simulink model "wlan_mac_hw"  (Simulink 7.8)
settings: Solver=ode45  StartTime=0.0  StopTime=200  RelTol=1e-3
PostLoadFcn:
  | wlan_mac_hw_init
InitFcn:
  | wlan_mac_hw_init
StartFcn:
  | wlan_mac_hw_init
values from neighbouring files (symbols this model uses):
  NB_CNTR_NAV = ceil(log2(MAX_NAV * 160))    [wlan_mac_hw_init.m]
  ticks_per_usec = 10    [wlan_mac_hw_init.m]
undefined symbols (not defined in the file or in its folder): gcbh, xlBlockLoadCallback, xlGetNormalizedPeriod
libraries: xbsIndex_r4 x788, xbsEDKLib_r4 x1
(part 5 of 6)

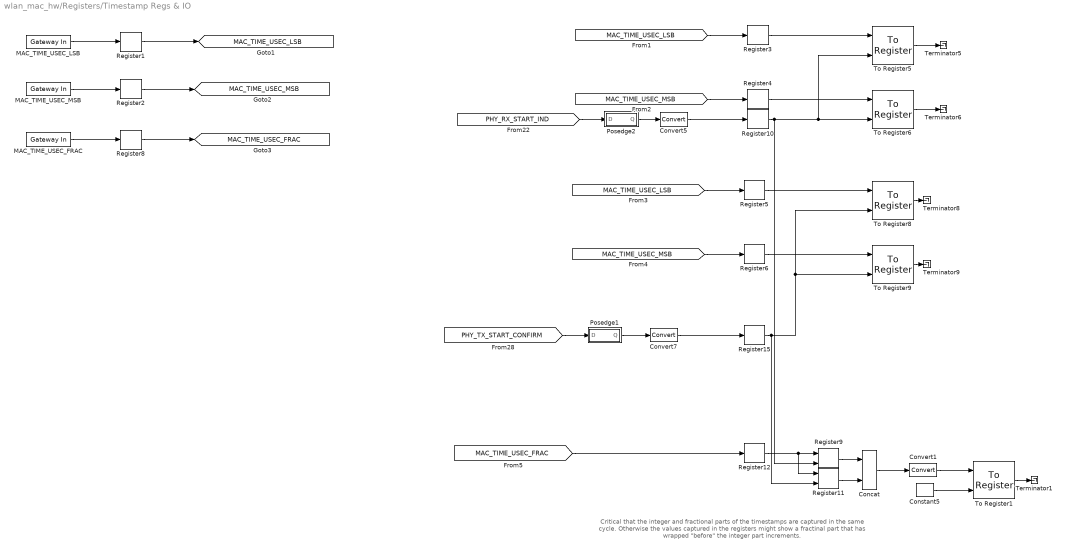
== system wlan_mac_hw/Registers/Timestamp Regs & IO ==
  note: Critical that the integer and fractional parts of the timestamps
      | are captured in the same cycle. Otherwise the values captured in the registers
      | might show a fractinal part that has wrapped "before" the integer part
      | increments.
  Concat : xbsIndex_r4/Concat  num_inputs=2  dbl_ovrd=off  block_type=concat
  Constant5 : xbsIndex_r4/Constant  const=1  gui_display_data_type=Boolean  arith_type=Boolean  n_bits=30  bin_pt=0  preci_type=Single  exp_width=8  frac_width=24  explicit_period=on  period=1  equ=P=C  opselect=C  inp2=PCIN>>17  opr=+  inp1=P  carry=CIN  dbl_ovrd=off  block_type=constant
  Convert1 : xbsIndex_r4/Convert  gui_display_data_type=Fixed-point  arith_type=Unsigned  n_bits=32  bin_pt=0  float_type=Single  exp_bits=8  fraction_bits=24  quantization=Truncate  overflow=Wrap  en=off  latency=0  dbl_ovrd=off  pipeline=off  block_type=convert
  Convert5 : xbsIndex_r4/Convert  gui_display_data_type=Boolean  arith_type=Boolean  n_bits=32  bin_pt=0  float_type=Single  exp_bits=8  fraction_bits=24  quantization=Truncate  overflow=Wrap  en=off  latency=0  dbl_ovrd=off  pipeline=off  block_type=convert
  Convert7 : xbsIndex_r4/Convert  gui_display_data_type=Boolean  arith_type=Boolean  n_bits=32  bin_pt=0  float_type=Single  exp_bits=8  fraction_bits=24  quantization=Truncate  overflow=Wrap  en=off  latency=0  dbl_ovrd=off  pipeline=off  block_type=convert
  MAC_TIME_USEC_FRAC : xbsIndex_r4/Gateway In  gui_display_data_type=Fixed-point  arith_type=Unsigned  n_bits=8  bin_pt=0  preci_type=Single  exp_width=8  frac_width=24  quantization="Round  (unbiased: +/- Inf)"  overflow=Saturate  period=1  dbl_ovrd=off  timing_constraint=None  locs_specified=off  LOCs={}  UseAsADC=off  ADCChannel='1'  inherit_from_input=off  hdl_port=on  block_type=gatewayin
  MAC_TIME_USEC_LSB : xbsIndex_r4/Gateway In  gui_display_data_type=Fixed-point  arith_type=Unsigned  n_bits=32  bin_pt=0  preci_type=Single  exp_width=8  frac_width=24  quantization="Round  (unbiased: +/- Inf)"  overflow=Saturate  period=1  dbl_ovrd=off  timing_constraint=None  locs_specified=off  LOCs={}  UseAsADC=off  ADCChannel='1'  inherit_from_input=off  hdl_port=on  block_type=gatewayin
  MAC_TIME_USEC_MSB : xbsIndex_r4/Gateway In  gui_display_data_type=Fixed-point  arith_type=Unsigned  n_bits=32  bin_pt=0  preci_type=Single  exp_width=8  frac_width=24  quantization="Round  (unbiased: +/- Inf)"  overflow=Saturate  period=1  dbl_ovrd=off  timing_constraint=None  locs_specified=off  LOCs={}  UseAsADC=off  ADCChannel='1'  inherit_from_input=off  hdl_port=on  block_type=gatewayin
  Posedge1 : Subsystem
  Posedge2 : Subsystem
  Register{1..6,8,10,12,15} (10 alike) : xbsIndex_r4/Register  init=0  rst=off  en=off  dbl_ovrd=off  block_type=register
  Register11 : xbsIndex_r4/Register  init=0  rst=off  en=on  dbl_ovrd=off  block_type=register
  Register9 : xbsIndex_r4/Register  init=0  rst=off  en=on  dbl_ovrd=off  block_type=register
  Terminator{1,5..6,8..9} (5 alike) : Terminator
  To Register1 : xbsIndex_r4/To Register  shared_memory_name='TXRX_START_TIMESTAMPS_FRAC'  init=0  ownership=Locally owned and initialized  explicit_data_type=on  gui_display_data_type=Fixed-point  arith_type=Unsigned  n_bits=32  bin_pt=0  preci_type=Single  dbl_ovrd=off  block_type=toreg
      settings: AttributesFormatString=<< %<shared_memory_name> >>  infoedit="Register block that writes data to a shared memory register.  Delay of one sample period."
  To Register5 : xbsIndex_r4/To Register  shared_memory_name='RX_START_TIMESTAMP_LSB'  init=0  ownership=Locally owned and initialized  explicit_data_type=on  gui_display_data_type=Fixed-point  arith_type=Unsigned  n_bits=32  bin_pt=0  preci_type=Single  dbl_ovrd=off  block_type=toreg
      settings: AttributesFormatString=<< %<shared_memory_name> >>  infoedit="Register block that writes data to a shared memory register.  Delay of one sample period."
  To Register6 : xbsIndex_r4/To Register  shared_memory_name='RX_START_TIMESTAMP_MSB'  init=0  ownership=Locally owned and initialized  explicit_data_type=on  gui_display_data_type=Fixed-point  arith_type=Unsigned  n_bits=32  bin_pt=0  preci_type=Single  dbl_ovrd=off  block_type=toreg
      settings: AttributesFormatString=<< %<shared_memory_name> >>  infoedit="Register block that writes data to a shared memory register.  Delay of one sample period."
  To Register8 : xbsIndex_r4/To Register  shared_memory_name='TX_START_TIMESTAMP_LSB'  init=0  ownership=Locally owned and initialized  explicit_data_type=on  gui_display_data_type=Fixed-point  arith_type=Unsigned  n_bits=32  bin_pt=0  preci_type=Single  dbl_ovrd=off  block_type=toreg
      settings: AttributesFormatString=<< %<shared_memory_name> >>  infoedit="Register block that writes data to a shared memory register.  Delay of one sample period."
  To Register9 : xbsIndex_r4/To Register  shared_memory_name='TX_START_TIMESTAMP_MSB'  init=0  ownership=Locally owned and initialized  explicit_data_type=on  gui_display_data_type=Fixed-point  arith_type=Unsigned  n_bits=32  bin_pt=0  preci_type=Single  dbl_ovrd=off  block_type=toreg
      settings: AttributesFormatString=<< %<shared_memory_name> >>  infoedit="Register block that writes data to a shared memory register.  Delay of one sample period."
  tag scope: MAC_TIME_USEC_FRAC=global, MAC_TIME_USEC_LSB=global, MAC_TIME_USEC_MSB=global
  wires:
  [MAC_TIME_USEC_LSB] -> Register3/1
  [PHY_RX_START_IND] -> Posedge2/1(D)
  [MAC_TIME_USEC_MSB] -> Register4/1
  To Register5/1 -> Terminator5/1
  To Register6/1 -> Terminator6/1
  [PHY_TX_START_CONFIRM] -> Posedge1/1(D)
  To Register8/1 -> Terminator8/1
  To Register9/1 -> Terminator9/1
  Register15/1 -> Register11/2, To Register9/2, To Register8/2
  Posedge2/1(Q) -> Convert5/1
  Convert7/1 -> Register15/1
  MAC_TIME_USEC_LSB/1 -> Register1/1
  MAC_TIME_USEC_MSB/1 -> Register2/1
  Register1/1 -> [MAC_TIME_USEC_LSB]
  Register2/1 -> [MAC_TIME_USEC_MSB]
  Register3/1 -> To Register5/1
  Register4/1 -> To Register6/1
  Convert5/1 -> Register10/1
  [MAC_TIME_USEC_LSB] -> Register5/1
  [MAC_TIME_USEC_MSB] -> Register6/1
  Register5/1 -> To Register8/1
  Register6/1 -> To Register9/1
  Posedge1/1(Q) -> Convert7/1
  MAC_TIME_USEC_FRAC/1 -> Register8/1
  Register8/1 -> [MAC_TIME_USEC_FRAC]
  Concat/1 -> Convert1/1
  Register9/1 -> Concat/1
  Register11/1 -> Concat/2
  [MAC_TIME_USEC_FRAC] -> Register12/1
  Convert1/1 -> To Register1/1
  Constant5/1 -> To Register1/2
  To Register1/1 -> Terminator1/1
  Register10/1 -> To Register6/2, To Register5/2, Register9/2
  Register12/1 -> Register9/1, Register11/1

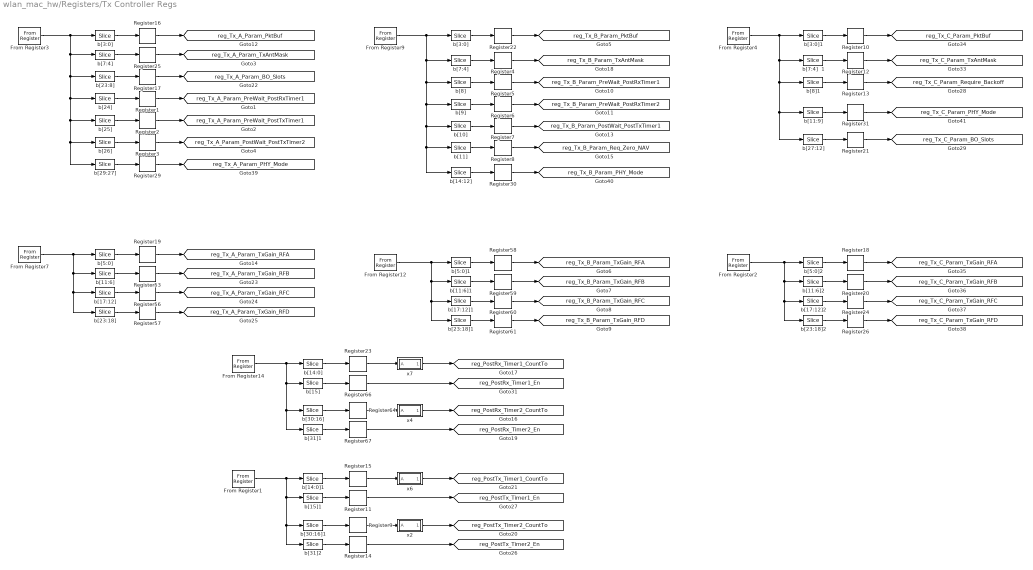
== system wlan_mac_hw/Registers/Tx Controller Regs ==
  " b[10]" : xbsIndex_r4/Slice  nbits=1  boolean_output=on  mode=Lower Bit Location + Width  bit1=0  base1=MSB of Input  bit0=10  base0=LSB of Input  dbl_ovrd=off  block_type=slice
      settings: block_version=VER_STRING_GOES_HERE
  " b[11:6]" : xbsIndex_r4/Slice  nbits=6  boolean_output=off  mode=Lower Bit Location + Width  bit1=0  base1=MSB of Input  bit0=6  base0=LSB of Input  dbl_ovrd=off  block_type=slice
      settings: block_version=VER_STRING_GOES_HERE
  " b[11:6]1" : xbsIndex_r4/Slice  nbits=6  boolean_output=off  mode=Lower Bit Location + Width  bit1=0  base1=MSB of Input  bit0=6  base0=LSB of Input  dbl_ovrd=off  block_type=slice
      settings: block_version=VER_STRING_GOES_HERE
  " b[11:6]2" : xbsIndex_r4/Slice  nbits=6  boolean_output=off  mode=Lower Bit Location + Width  bit1=0  base1=MSB of Input  bit0=6  base0=LSB of Input  dbl_ovrd=off  block_type=slice
      settings: block_version=VER_STRING_GOES_HERE
  " b[11:9]" : xbsIndex_r4/Slice  nbits=3  boolean_output=off  mode=Lower Bit Location + Width  bit1=0  base1=MSB of Input  bit0=9  base0=LSB of Input  dbl_ovrd=off  block_type=slice
      settings: block_version=VER_STRING_GOES_HERE
  " b[11]" : xbsIndex_r4/Slice  nbits=1  boolean_output=on  mode=Lower Bit Location + Width  bit1=0  base1=MSB of Input  bit0=11  base0=LSB of Input  dbl_ovrd=off  block_type=slice
      settings: block_version=VER_STRING_GOES_HERE
  " b[14:0]" : xbsIndex_r4/Slice  nbits=15  boolean_output=off  mode=Lower Bit Location + Width  bit1=0  base1=MSB of Input  bit0=0  base0=LSB of Input  dbl_ovrd=off  block_type=slice
      settings: block_version=VER_STRING_GOES_HERE
  " b[14:0]1" : xbsIndex_r4/Slice  nbits=15  boolean_output=off  mode=Lower Bit Location + Width  bit1=0  base1=MSB of Input  bit0=0  base0=LSB of Input  dbl_ovrd=off  block_type=slice
      settings: block_version=VER_STRING_GOES_HERE
  " b[14:12]" : xbsIndex_r4/Slice  nbits=3  boolean_output=off  mode=Lower Bit Location + Width  bit1=0  base1=MSB of Input  bit0=12  base0=LSB of Input  dbl_ovrd=off  block_type=slice
      settings: block_version=VER_STRING_GOES_HERE
  " b[15]" : xbsIndex_r4/Slice  nbits=1  boolean_output=on  mode=Lower Bit Location + Width  bit1=0  base1=MSB of Input  bit0=15  base0=LSB of Input  dbl_ovrd=off  block_type=slice
      settings: block_version=VER_STRING_GOES_HERE
  " b[15]1" : xbsIndex_r4/Slice  nbits=1  boolean_output=on  mode=Lower Bit Location + Width  bit1=0  base1=MSB of Input  bit0=15  base0=LSB of Input  dbl_ovrd=off  block_type=slice
      settings: block_version=VER_STRING_GOES_HERE
  " b[17:12]" : xbsIndex_r4/Slice  nbits=6  boolean_output=off  mode=Lower Bit Location + Width  bit1=0  base1=MSB of Input  bit0=12  base0=LSB of Input  dbl_ovrd=off  block_type=slice
      settings: block_version=VER_STRING_GOES_HERE
  " b[17:12]1" : xbsIndex_r4/Slice  nbits=6  boolean_output=off  mode=Lower Bit Location + Width  bit1=0  base1=MSB of Input  bit0=12  base0=LSB of Input  dbl_ovrd=off  block_type=slice
      settings: block_version=VER_STRING_GOES_HERE
  " b[17:12]2" : xbsIndex_r4/Slice  nbits=6  boolean_output=off  mode=Lower Bit Location + Width  bit1=0  base1=MSB of Input  bit0=12  base0=LSB of Input  dbl_ovrd=off  block_type=slice
      settings: block_version=VER_STRING_GOES_HERE
  " b[23:18]" : xbsIndex_r4/Slice  nbits=6  boolean_output=off  mode=Lower Bit Location + Width  bit1=0  base1=MSB of Input  bit0=18  base0=LSB of Input  dbl_ovrd=off  block_type=slice
      settings: block_version=VER_STRING_GOES_HERE
  " b[23:18]1" : xbsIndex_r4/Slice  nbits=6  boolean_output=off  mode=Lower Bit Location + Width  bit1=0  base1=MSB of Input  bit0=18  base0=LSB of Input  dbl_ovrd=off  block_type=slice
      settings: block_version=VER_STRING_GOES_HERE
  " b[23:18]2" : xbsIndex_r4/Slice  nbits=6  boolean_output=off  mode=Lower Bit Location + Width  bit1=0  base1=MSB of Input  bit0=18  base0=LSB of Input  dbl_ovrd=off  block_type=slice
      settings: block_version=VER_STRING_GOES_HERE
  " b[23:8]" : xbsIndex_r4/Slice  nbits=16  boolean_output=off  mode=Lower Bit Location + Width  bit1=0  base1=MSB of Input  bit0=8  base0=LSB of Input  dbl_ovrd=off  block_type=slice
      settings: block_version=VER_STRING_GOES_HERE
  " b[24]" : xbsIndex_r4/Slice  nbits=1  boolean_output=on  mode=Lower Bit Location + Width  bit1=0  base1=MSB of Input  bit0=24  base0=LSB of Input  dbl_ovrd=off  block_type=slice
      settings: block_version=VER_STRING_GOES_HERE
  " b[25]" : xbsIndex_r4/Slice  nbits=1  boolean_output=on  mode=Lower Bit Location + Width  bit1=0  base1=MSB of Input  bit0=25  base0=LSB of Input  dbl_ovrd=off  block_type=slice
      settings: block_version=VER_STRING_GOES_HERE
  " b[26]" : xbsIndex_r4/Slice  nbits=1  boolean_output=on  mode=Lower Bit Location + Width  bit1=0  base1=MSB of Input  bit0=26  base0=LSB of Input  dbl_ovrd=off  block_type=slice
      settings: block_version=VER_STRING_GOES_HERE
  " b[27:12]" : xbsIndex_r4/Slice  nbits=16  boolean_output=off  mode=Lower Bit Location + Width  bit1=0  base1=MSB of Input  bit0=12  base0=LSB of Input  dbl_ovrd=off  block_type=slice
      settings: block_version=VER_STRING_GOES_HERE
  " b[29:27]" : xbsIndex_r4/Slice  nbits=3  boolean_output=off  mode=Lower Bit Location + Width  bit1=0  base1=MSB of Input  bit0=27  base0=LSB of Input  dbl_ovrd=off  block_type=slice
      settings: block_version=VER_STRING_GOES_HERE
  " b[30:16]" : xbsIndex_r4/Slice  nbits=15  boolean_output=off  mode=Lower Bit Location + Width  bit1=0  base1=MSB of Input  bit0=16  base0=LSB of Input  dbl_ovrd=off  block_type=slice
      settings: block_version=VER_STRING_GOES_HERE
  " b[30:16]1" : xbsIndex_r4/Slice  nbits=15  boolean_output=off  mode=Lower Bit Location + Width  bit1=0  base1=MSB of Input  bit0=16  base0=LSB of Input  dbl_ovrd=off  block_type=slice
      settings: block_version=VER_STRING_GOES_HERE
  " b[31]1" : xbsIndex_r4/Slice  nbits=1  boolean_output=on  mode=Lower Bit Location + Width  bit1=0  base1=MSB of Input  bit0=31  base0=LSB of Input  dbl_ovrd=off  block_type=slice
      settings: block_version=VER_STRING_GOES_HERE
  " b[31]2" : xbsIndex_r4/Slice  nbits=1  boolean_output=on  mode=Lower Bit Location + Width  bit1=0  base1=MSB of Input  bit0=31  base0=LSB of Input  dbl_ovrd=off  block_type=slice
      settings: block_version=VER_STRING_GOES_HERE
  " b[3:0]" : xbsIndex_r4/Slice  nbits=4  boolean_output=off  mode=Lower Bit Location + Width  bit1=0  base1=MSB of Input  bit0=0  base0=LSB of Input  dbl_ovrd=off  block_type=slice
      settings: block_version=VER_STRING_GOES_HERE
  " b[3:0] " : xbsIndex_r4/Slice  nbits=4  boolean_output=off  mode=Lower Bit Location + Width  bit1=0  base1=MSB of Input  bit0=0  base0=LSB of Input  dbl_ovrd=off  block_type=slice
      settings: block_version=VER_STRING_GOES_HERE
  " b[3:0]1" : xbsIndex_r4/Slice  nbits=4  boolean_output=off  mode=Lower Bit Location + Width  bit1=0  base1=MSB of Input  bit0=0  base0=LSB of Input  dbl_ovrd=off  block_type=slice
      settings: block_version=VER_STRING_GOES_HERE
  " b[5:0]" : xbsIndex_r4/Slice  nbits=6  boolean_output=off  mode=Lower Bit Location + Width  bit1=0  base1=MSB of Input  bit0=0  base0=LSB of Input  dbl_ovrd=off  block_type=slice
      settings: block_version=VER_STRING_GOES_HERE
  " b[5:0]1" : xbsIndex_r4/Slice  nbits=6  boolean_output=off  mode=Lower Bit Location + Width  bit1=0  base1=MSB of Input  bit0=0  base0=LSB of Input  dbl_ovrd=off  block_type=slice
      settings: block_version=VER_STRING_GOES_HERE
  " b[5:0]2" : xbsIndex_r4/Slice  nbits=6  boolean_output=off  mode=Lower Bit Location + Width  bit1=0  base1=MSB of Input  bit0=0  base0=LSB of Input  dbl_ovrd=off  block_type=slice
      settings: block_version=VER_STRING_GOES_HERE
  " b[7:4]" : xbsIndex_r4/Slice  nbits=4  boolean_output=off  mode=Lower Bit Location + Width  bit1=0  base1=MSB of Input  bit0=4  base0=LSB of Input  dbl_ovrd=off  block_type=slice
      settings: block_version=VER_STRING_GOES_HERE
  " b[7:4]  " : xbsIndex_r4/Slice  nbits=4  boolean_output=off  mode=Lower Bit Location + Width  bit1=0  base1=MSB of Input  bit0=4  base0=LSB of Input  dbl_ovrd=off  block_type=slice
      settings: block_version=VER_STRING_GOES_HERE
  " b[7:4]  1" : xbsIndex_r4/Slice  nbits=4  boolean_output=off  mode=Lower Bit Location + Width  bit1=0  base1=MSB of Input  bit0=4  base0=LSB of Input  dbl_ovrd=off  block_type=slice
      settings: block_version=VER_STRING_GOES_HERE
  " b[8]" : xbsIndex_r4/Slice  nbits=1  boolean_output=on  mode=Lower Bit Location + Width  bit1=0  base1=MSB of Input  bit0=8  base0=LSB of Input  dbl_ovrd=off  block_type=slice
      settings: block_version=VER_STRING_GOES_HERE
  " b[8]1" : xbsIndex_r4/Slice  nbits=1  boolean_output=on  mode=Lower Bit Location + Width  bit1=0  base1=MSB of Input  bit0=8  base0=LSB of Input  dbl_ovrd=off  block_type=slice
      settings: block_version=VER_STRING_GOES_HERE
  " b[9]" : xbsIndex_r4/Slice  nbits=1  boolean_output=on  mode=Lower Bit Location + Width  bit1=0  base1=MSB of Input  bit0=9  base0=LSB of Input  dbl_ovrd=off  block_type=slice
      settings: block_version=VER_STRING_GOES_HERE
  From Register1 : xbsIndex_r4/From Register  shared_memory_name='POST_TX_TIMERS'  init=REG_MAC_PostTxTimers  period=1  ownership=Locally owned and initialized  gui_display_data_type=Fixed-point  arith_type=Unsigned  n_bits=32  bin_pt=0  preci_type=Single  dbl_ovrd=off  block_type=fromreg
      settings: AttributesFormatString=<< %<shared_memory_name> >>  infoedit="Register block that reads data to a shared memory register.  Delay of one sample period."
  From Register12 : xbsIndex_r4/From Register  shared_memory_name='TX_CTRL_B_GAINS'  init=0  period=1  ownership=Locally owned and initialized  gui_display_data_type=Fixed-point  arith_type=Unsigned  n_bits=32  bin_pt=0  preci_type=Single  dbl_ovrd=off  block_type=fromreg
      settings: AttributesFormatString=<< %<shared_memory_name> >>  infoedit="Register block that reads data to a shared memory register.  Delay of one sample period."
  From Register14 : xbsIndex_r4/From Register  shared_memory_name='POST_RX_TIMERS'  init=REG_MAC_PostRxTimers  period=1  ownership=Locally owned and initialized  gui_display_data_type=Fixed-point  arith_type=Unsigned  n_bits=32  bin_pt=0  preci_type=Single  dbl_ovrd=off  block_type=fromreg
      settings: AttributesFormatString=<< %<shared_memory_name> >>  infoedit="Register block that reads data to a shared memory register.  Delay of one sample period."
  From Register2 : xbsIndex_r4/From Register  shared_memory_name='TX_CTRL_C_GAINS'  init=0  period=1  ownership=Locally owned and initialized  gui_display_data_type=Fixed-point  arith_type=Unsigned  n_bits=32  bin_pt=0  preci_type=Single  dbl_ovrd=off  block_type=fromreg
      settings: AttributesFormatString=<< %<shared_memory_name> >>  infoedit="Register block that reads data to a shared memory register.  Delay of one sample period."
  From Register3 : xbsIndex_r4/From Register  shared_memory_name='TX_CTRL_A_PARAMS'  init=REG_MAC_Tx_Ctrl_A_Params  period=1  ownership=Locally owned and initialized  gui_display_data_type=Fixed-point  arith_type=Unsigned  n_bits=32  bin_pt=0  preci_type=Single  dbl_ovrd=off  block_type=fromreg
      settings: AttributesFormatString=<< %<shared_memory_name> >>  infoedit="Register block that reads data to a shared memory register.  Delay of one sample period."
  From Register4 : xbsIndex_r4/From Register  shared_memory_name='TX_CTRL_C_PARAMS'  init=REG_MAC_Tx_Ctrl_C_Params  period=1  ownership=Locally owned and initialized  gui_display_data_type=Fixed-point  arith_type=Unsigned  n_bits=32  bin_pt=0  preci_type=Single  dbl_ovrd=off  block_type=fromreg
      settings: AttributesFormatString=<< %<shared_memory_name> >>  infoedit="Register block that reads data to a shared memory register.  Delay of one sample period."
  From Register7 : xbsIndex_r4/From Register  shared_memory_name='TX_CTRL_A_GAINS'  init=0  period=1  ownership=Locally owned and initialized  gui_display_data_type=Fixed-point  arith_type=Unsigned  n_bits=32  bin_pt=0  preci_type=Single  dbl_ovrd=off  block_type=fromreg
      settings: AttributesFormatString=<< %<shared_memory_name> >>  infoedit="Register block that reads data to a shared memory register.  Delay of one sample period."
  From Register9 : xbsIndex_r4/From Register  shared_memory_name='TX_CTRL_B_PARAMS'  init=REG_MAC_Tx_Ctrl_B_Params  period=1  ownership=Locally owned and initialized  gui_display_data_type=Fixed-point  arith_type=Unsigned  n_bits=32  bin_pt=0  preci_type=Single  dbl_ovrd=off  block_type=fromreg
      settings: AttributesFormatString=<< %<shared_memory_name> >>  infoedit="Register block that reads data to a shared memory register.  Delay of one sample period."
  Register{1..26,29..31,53,56..61,64,66..67} (39 alike) : xbsIndex_r4/Register  init=0  rst=off  en=off  dbl_ovrd=off  block_type=register
  x2 : Subsystem
  x4 : Subsystem
  x6 : Subsystem
  x7 : Subsystem
  tag scope: reg_PostRx_Timer1_CountTo=global, reg_PostRx_Timer1_En=global, reg_PostRx_Timer2_CountTo=global, reg_PostRx_Timer2_En=global, reg_PostTx_Timer1_CountTo=global, reg_PostTx_Timer1_En=global, reg_PostTx_Timer2_CountTo=global, reg_PostTx_Timer2_En=global, reg_Tx_A_Param_BO_Slots=global, reg_Tx_A_Param_PHY_Mode=global, reg_Tx_A_Param_PktBuf=global, reg_Tx_A_Param_PostWait_PostTxTimer2=global, reg_Tx_A_Param_PreWait_PostRxTimer1=global, reg_Tx_A_Param_PreWait_PostTxTimer1=global, reg_Tx_A_Param_TxAntMask=global, reg_Tx_A_Param_TxGain_RFA=global, reg_Tx_A_Param_TxGain_RFB=global, reg_Tx_A_Param_TxGain_RFC=global, reg_Tx_A_Param_TxGain_RFD=global, reg_Tx_B_Param_PHY_Mode=global, reg_Tx_B_Param_PktBuf=global, reg_Tx_B_Param_PostWait_PostTxTimer1=global, reg_Tx_B_Param_PreWait_PostRxTimer1=global, reg_Tx_B_Param_PreWait_PostRxTimer2=global, reg_Tx_B_Param_Req_Zero_NAV=global, reg_Tx_B_Param_TxAntMask=global, reg_Tx_B_Param_TxGain_RFA=global, reg_Tx_B_Param_TxGain_RFB=global, reg_Tx_B_Param_TxGain_RFC=global, reg_Tx_B_Param_TxGain_RFD=global, reg_Tx_C_Param_BO_Slots=global, reg_Tx_C_Param_PHY_Mode=global, reg_Tx_C_Param_PktBuf=global, reg_Tx_C_Param_Require_Backoff=global, reg_Tx_C_Param_TxAntMask=global, reg_Tx_C_Param_TxGain_RFA=global, reg_Tx_C_Param_TxGain_RFB=global, reg_Tx_C_Param_TxGain_RFC=global, reg_Tx_C_Param_TxGain_RFD=global
  wires:
  From Register3/1 -> " b[3:0] "/1, " b[7:4]"/1, " b[23:8]"/1, " b[24]"/1, " b[25]"/1, " b[26]"/1, " b[29:27]"/1
  From Register9/1 -> " b[3:0]"/1, " b[7:4]  "/1, " b[8]"/1, " b[10]"/1, " b[11]"/1, " b[14:12]"/1, " b[9]"/1
  " b[3:0]"/1 -> Register22/1
  " b[3:0] "/1 -> Register16/1
  " b[23:8]"/1 -> Register17/1
  " b[5:0]"/1 -> Register19/1
  Register16/1 -> [reg_Tx_A_Param_PktBuf]
  Register17/1 -> [reg_Tx_A_Param_BO_Slots]
  Register19/1 -> [reg_Tx_A_Param_TxGain_RFA]
  Register22/1 -> [reg_Tx_B_Param_PktBuf]
  " b[7:4]"/1 -> Register25/1
  Register25/1 -> [reg_Tx_A_Param_TxAntMask]
  " b[7:4]  "/1 -> Register4/1
  From Register7/1 -> " b[5:0]"/1, " b[11:6]"/1, " b[17:12]"/1, " b[23:18]"/1
  " b[11:6]"/1 -> Register53/1
  " b[17:12]"/1 -> Register56/1
  " b[23:18]"/1 -> Register57/1
  Register53/1 -> [reg_Tx_A_Param_TxGain_RFB]
  Register56/1 -> [reg_Tx_A_Param_TxGain_RFC]
  Register57/1 -> [reg_Tx_A_Param_TxGain_RFD]
  " b[24]"/1 -> Register1/1
  " b[25]"/1 -> Register2/1
  " b[26]"/1 -> Register3/1
  Register1/1 -> [reg_Tx_A_Param_PreWait_PostRxTimer1]
  Register2/1 -> [reg_Tx_A_Param_PreWait_PostTxTimer1]
  Register3/1 -> [reg_Tx_A_Param_PostWait_PostTxTimer2]
  " b[8]"/1 -> Register5/1
  " b[9]"/1 -> Register6/1
  " b[10]"/1 -> Register7/1
  " b[11]"/1 -> Register8/1
  " b[5:0]1"/1 -> Register58/1
  Register58/1 -> [reg_Tx_B_Param_TxGain_RFA]
  From Register12/1 -> " b[5:0]1"/1, " b[11:6]1"/1, " b[17:12]1"/1, " b[23:18]1"/1
  " b[11:6]1"/1 -> Register59/1
  " b[17:12]1"/1 -> Register60/1
  " b[23:18]1"/1 -> Register61/1
  Register59/1 -> [reg_Tx_B_Param_TxGain_RFB]
  Register60/1 -> [reg_Tx_B_Param_TxGain_RFC]
  Register61/1 -> [reg_Tx_B_Param_TxGain_RFD]
  Register4/1 -> [reg_Tx_B_Param_TxAntMask]
  Register5/1 -> [reg_Tx_B_Param_PreWait_PostRxTimer1]
  Register6/1 -> [reg_Tx_B_Param_PreWait_PostRxTimer2]
  Register7/1 -> [reg_Tx_B_Param_PostWait_PostTxTimer1]
  Register8/1 -> [reg_Tx_B_Param_Req_Zero_NAV]
  " b[14:0]"/1 -> Register23/1
  x7/1(Ax16) -> [reg_PostRx_Timer1_CountTo]
  Register23/1 -> x7/1(A)
  Register66/1 -> [reg_PostRx_Timer1_En]
  " b[15]"/1 -> Register66/1
  " b[30:16]"/1 -> Register64/1
  x4/1(Ax16) -> [reg_PostRx_Timer2_CountTo]
  Register64/1 -> x4/1(A)
  Register67/1 -> [reg_PostRx_Timer2_En]
  " b[31]1"/1 -> Register67/1
  From Register14/1 -> " b[14:0]"/1, " b[15]"/1, " b[30:16]"/1, " b[31]1"/1
  " b[14:0]1"/1 -> Register15/1
  x6/1(Ax16) -> [reg_PostTx_Timer1_CountTo]
  Register15/1 -> x6/1(A)
  Register11/1 -> [reg_PostTx_Timer1_En]
  " b[15]1"/1 -> Register11/1
  " b[30:16]1"/1 -> Register9/1
  x2/1(Ax16) -> [reg_PostTx_Timer2_CountTo]
  Register9/1 -> x2/1(A)
  Register14/1 -> [reg_PostTx_Timer2_En]
  " b[31]2"/1 -> Register14/1
  From Register1/1 -> " b[31]2"/1, " b[30:16]1"/1, " b[15]1"/1, " b[14:0]1"/1
  From Register4/1 -> " b[8]1"/1, " b[11:9]"/1, " b[27:12]"/1, " b[7:4]  1"/1, " b[3:0]1"/1
  " b[3:0]1"/1 -> Register10/1
  Register10/1 -> [reg_Tx_C_Param_PktBuf]
  " b[7:4]  1"/1 -> Register12/1
  " b[8]1"/1 -> Register13/1
  " b[5:0]2"/1 -> Register18/1
  Register18/1 -> [reg_Tx_C_Param_TxGain_RFA]
  From Register2/1 -> " b[23:18]2"/1, " b[17:12]2"/1, " b[11:6]2"/1, " b[5:0]2"/1
  " b[11:6]2"/1 -> Register20/1
  " b[17:12]2"/1 -> Register24/1
  " b[23:18]2"/1 -> Register26/1
  Register20/1 -> [reg_Tx_C_Param_TxGain_RFB]
  Register24/1 -> [reg_Tx_C_Param_TxGain_RFC]
  Register26/1 -> [reg_Tx_C_Param_TxGain_RFD]
  Register12/1 -> [reg_Tx_C_Param_TxAntMask]
  Register13/1 -> [reg_Tx_C_Param_Require_Backoff]
  " b[29:27]"/1 -> Register29/1
  Register29/1 -> [reg_Tx_A_Param_PHY_Mode]
  " b[14:12]"/1 -> Register30/1
  Register30/1 -> [reg_Tx_B_Param_PHY_Mode]
  " b[11:9]"/1 -> Register31/1
  Register31/1 -> [reg_Tx_C_Param_PHY_Mode]
  " b[27:12]"/1 -> Register21/1
  Register21/1 -> [reg_Tx_C_Param_BO_Slots]

== system wlan_mac_hw/Registers/x1 ==
  A : Inport
  Concat1 : xbsIndex_r4/Concat  num_inputs=2  dbl_ovrd=off  block_type=concat
  Constant9 : xbsIndex_r4/Constant  const=0  gui_display_data_type=Fixed-point  arith_type=Unsigned  n_bits=4  bin_pt=0  preci_type=Single  exp_width=8  frac_width=24  explicit_period=off  period=1  equ=P=C  opselect=C  inp2=PCIN>>17  opr=+  inp1=P  carry=CIN  dbl_ovrd=off  block_type=constant
  Ax16 : Outport
  wires:
  Concat1/1 -> Ax16/1
  A/1 -> Concat1/1
  Constant9/1 -> Concat1/2

== system wlan_mac_hw/Registers/x16 ==
  A : Inport
  Concat1 : xbsIndex_r4/Concat  num_inputs=2  dbl_ovrd=off  block_type=concat
  Constant9 : xbsIndex_r4/Constant  const=0  gui_display_data_type=Fixed-point  arith_type=Unsigned  n_bits=4  bin_pt=0  preci_type=Single  exp_width=8  frac_width=24  explicit_period=off  period=1  equ=P=C  opselect=C  inp2=PCIN>>17  opr=+  inp1=P  carry=CIN  dbl_ovrd=off  block_type=constant
  Ax16 : Outport
  wires:
  Constant9/1 -> Concat1/2
  A/1 -> Concat1/1
  Concat1/1 -> Ax16/1

== system wlan_mac_hw/Registers/x3 ==
  A : Inport
  Concat1 : xbsIndex_r4/Concat  num_inputs=2  dbl_ovrd=off  block_type=concat
  Constant9 : xbsIndex_r4/Constant  const=0  gui_display_data_type=Fixed-point  arith_type=Unsigned  n_bits=4  bin_pt=0  preci_type=Single  exp_width=8  frac_width=24  explicit_period=off  period=1  equ=P=C  opselect=C  inp2=PCIN>>17  opr=+  inp1=P  carry=CIN  dbl_ovrd=off  block_type=constant
  Ax16 : Outport
  wires:
  Concat1/1 -> Ax16/1
  A/1 -> Concat1/1
  Constant9/1 -> Concat1/2

== system wlan_mac_hw/Registers/x5 ==
  A : Inport
  Concat1 : xbsIndex_r4/Concat  num_inputs=2  dbl_ovrd=off  block_type=concat
  Constant9 : xbsIndex_r4/Constant  const=0  gui_display_data_type=Fixed-point  arith_type=Unsigned  n_bits=4  bin_pt=0  preci_type=Single  exp_width=8  frac_width=24  explicit_period=off  period=1  equ=P=C  opselect=C  inp2=PCIN>>17  opr=+  inp1=P  carry=CIN  dbl_ovrd=off  block_type=constant
  Ax16 : Outport
  wires:
  Constant9/1 -> Concat1/2
  A/1 -> Concat1/1
  Concat1/1 -> Ax16/1

== system wlan_mac_hw/Registers/x8 ==
  A : Inport
  Concat1 : xbsIndex_r4/Concat  num_inputs=2  dbl_ovrd=off  block_type=concat
  Constant9 : xbsIndex_r4/Constant  const=0  gui_display_data_type=Fixed-point  arith_type=Unsigned  n_bits=4  bin_pt=0  preci_type=Single  exp_width=8  frac_width=24  explicit_period=off  period=1  equ=P=C  opselect=C  inp2=PCIN>>17  opr=+  inp1=P  carry=CIN  dbl_ovrd=off  block_type=constant
  Ax16 : Outport
  wires:
  Concat1/1 -> Ax16/1
  A/1 -> Concat1/1
  Constant9/1 -> Concat1/2

== system wlan_mac_hw/Slot Time/Posedge2 ==
  note: Rising Edge Detection
  D : Inport
  Delay : xbsIndex_r4/Delay  rst=off  infoeditControl=Selection of Reset will increase slice count due to use of real FFs and instead of SRLs  en=off  latency=1  dbl_ovrd=off  reg_retiming=off  block_type=delay
      settings: infoedit=Hardware notes: A delay line is a chain, each link of which is an SRL16 followed by a flip-flop. If register retiming is enabled, the delay line is a chain of flip-flops.  xl_area=[1 1 0 0 0 0 0]  block_version=VER_STRING_GOES_HERE
  Inverter : xbsIndex_r4/Inverter  en=off  latency=0  dbl_ovrd=off  block_type=inv
      settings: xl_area=[0 0 0 0 0 0 0]  block_version=VER_STRING_GOES_HERE
  Logical1 : xbsIndex_r4/Logical  logical_function=AND  inputs=2  en=off  latency=0  precision=Full  arith_type=Unsigned  n_bits=8  bin_pt=2  align_bp=on  dbl_ovrd=off  block_type=logical
      settings: xl_area=[1 0 0 1 0 0 0]  block_version=VER_STRING_GOES_HERE
  Q : Outport
  wires:
  D/1 -> Logical1/2, Delay/1
  Logical1/1 -> Q/1
  Inverter/1 -> Logical1/1
  Delay/1 -> Inverter/1

== system wlan_mac_hw/TBTT/S-R Latch1 ==
  S : Inport
  R : Inport  Port=2
  Constant1 : xbsIndex_r4/Constant  const=1  gui_display_data_type=Boolean  arith_type=Boolean  n_bits=1  bin_pt=0  preci_type=Single  exp_width=8  frac_width=24  explicit_period=off  period=1  equ=P=C  opselect=C  inp2=PCIN>>17  opr=+  inp1=P  carry=CIN  dbl_ovrd=off  block_type=constant
      settings: block_version=VER_STRING_GOES_HERE
  Register2 : xbsIndex_r4/Register  init=0  rst=on  en=on  dbl_ovrd=off  block_type=register
      settings: xl_area=[1 1 0 0 0 0 0]  block_version=VER_STRING_GOES_HERE
  Q : Outport
  wires:
  S/1 -> Register2/3
  Register2/1 -> Q/1
  R/1 -> Register2/2
  Constant1/1 -> Register2/1

== system wlan_mac_hw/Tx Control A/A Backoff ==
  note: Sanity Checks:
      | Assuming IDLE_FOR_DIFS asserts and stays high.
      |
      | If NUM_BO_SLOTS = 0, core should transmit when BACKOFF_START asserts with no extra waiting
      |
      | If NUM_BO_SLOTS = 1, core should transmit exactly 1 slot time after BACKOFF_START asserts
  note: Software-initiated backoff gets priority
      | But any "start backoff" is ignored if a
      | previous backoff is still active.
  note: Backoff decrements on slot boundary only
      | if Tx C is not pending. This implements the
      | spec's requirement of suspending backoff of
      | current Tx when transmitting beacon at TBTT.
      |
      | Current hardware path of Tx_C==PENDING has
      | narrow race window, when Tx A is transitioning from
      | DEFER to DO_TX. The software-set backoff pause
      | bit above allows an all-software Tx C if-not Tx A.
      | We'll try both in hardware and see works better.
  Backoff : Scope  NumInputPorts=5
      settings: YMin=-1~0.95~0.95~-5~-5  YMax=1~1.05~1.05~5~5
  Constant : xbsIndex_r4/Constant  const=0  gui_display_data_type=Fixed-point  arith_type=Unsigned  n_bits=1  bin_pt=0  preci_type=Single  exp_width=8  frac_width=24  explicit_period=off  period=1  equ=P=C  opselect=C  inp2=PCIN>>17  opr=+  inp1=P  carry=CIN  dbl_ovrd=off  block_type=constant
  Convert : xbsIndex_r4/Convert  gui_display_data_type=Fixed-point  arith_type=Unsigned  n_bits=NB_CNTR_NUM_SLOTS  bin_pt=0  float_type=Single  exp_bits=8  fraction_bits=24  quantization=Truncate  overflow=Wrap  en=off  latency=0  dbl_ovrd=off  pipeline=off  block_type=convert
  Ctrl : Subsystem
  Gateway Out{,1..4} (5 alike) : xbsIndex_r4/Gateway Out  inherit_from_input=off  hdl_port=off  timing_constraint=None  locs_specified=off  LOCs={}  UseAsDAC=off  DACChannel='1'  block_type=gatewayout
  Inverter : xbsIndex_r4/Inverter  en=off  latency=0  dbl_ovrd=off  block_type=inv
      settings: xl_area=[0 0 0 0 0 0 0]  block_version=VER_STRING_GOES_HERE
  Inverter1 : xbsIndex_r4/Inverter  en=off  latency=0  dbl_ovrd=off  block_type=inv
      settings: xl_area=[0 0 0 0 0 0 0]  block_version=VER_STRING_GOES_HERE
  Inverter2 : xbsIndex_r4/Inverter  en=off  latency=0  dbl_ovrd=off  block_type=inv
      settings: xl_area=[0 0 0 0 0 0 0]  block_version=VER_STRING_GOES_HERE
  Logical1 : xbsIndex_r4/Logical  logical_function=AND  inputs=4  en=off  latency=0  precision=Full  arith_type=Unsigned  n_bits=16  bin_pt=0  align_bp=on  dbl_ovrd=off  block_type=logical
  Logical2 : xbsIndex_r4/Logical  logical_function=OR  inputs=2  en=off  latency=0  precision=Full  arith_type=Unsigned  n_bits=16  bin_pt=0  align_bp=on  dbl_ovrd=off  block_type=logical
  Logical3 : xbsIndex_r4/Logical  logical_function=OR  inputs=2  en=off  latency=0  precision=Full  arith_type=Unsigned  n_bits=16  bin_pt=0  align_bp=on  dbl_ovrd=off  block_type=logical
  Logical6 : xbsIndex_r4/Logical  logical_function=OR  inputs=2  en=off  latency=0  precision=Full  arith_type=Unsigned  n_bits=16  bin_pt=0  align_bp=on  dbl_ovrd=off  block_type=logical
  Mux : xbsIndex_r4/Mux  inputs=2  en=off  latency=0  precision=Full  arith_type=Unsigned  n_bits=16  bin_pt=14  quantization=Truncate  overflow=Wrap  dbl_ovrd=off  block_type=mux
  Num Slots : xbsIndex_r4/Counter  cnt_type=Free Running  cnt_to=0  operation=Down  start_count=0  cnt_by_val=1  arith_type=Unsigned  n_bits=NB_CNTR_NUM_SLOTS  bin_pt=0  load_pin=on  rst=on  en=on  explicit_period=off  period=1  dbl_ovrd=off  use_behavioral_HDL=off  implementation=Fabric  block_type=counter
  Register : xbsIndex_r4/Register  init=0  rst=off  en=off  dbl_ovrd=off  block_type=register
  Register1 : xbsIndex_r4/Register  init=0  rst=off  en=off  dbl_ovrd=off  block_type=register
  Register2 : xbsIndex_r4/Register  init=0  rst=off  en=on  dbl_ovrd=off  block_type=register
      settings: xl_area=[1 1 0 0 0 0 0]  block_version=VER_STRING_GOES_HERE
  Relational1 : xbsIndex_r4/Relational  mode=a=b  en=off  latency=0  dbl_ovrd=off  block_type=relational
  dbg_Backoff_A_active : xbsIndex_r4/Gateway Out  inherit_from_input=off  hdl_port=on  timing_constraint=None  locs_specified=off  LOCs={}  UseAsDAC=off  DACChannel='1'  block_type=gatewayout
  Backoff Done : Outport
  tag scope: Status_Current_A_Backoff_Count=global
  wires:
  Convert/1 -> Num Slots/2
  [IDLE_FOR_TXDIFS] -> Ctrl/4(Idle for DIFS), Gateway Out2/1
  Constant/1 -> Relational1/2
  Relational1/1 -> Inverter/1, Ctrl/1(BO Zero)
  Num Slots/1 -> Relational1/1, [Status_Current_A_Backoff_Count], Gateway Out4/1
  [Tx_A_Num_BO_Slots] -> Mux/2
  [reg_Backoff_Sw_NumSlots] -> Mux/3
  [reg_Backoff_Sw_Start] -> Mux/1, Logical6/2
  Mux/1 -> Register2/1, Ctrl/3(Num Slots)
  Register2/1 -> Convert/1
  Logical6/1 -> Register2/2, Gateway Out/1, Ctrl/2(BO Start)
  [Tx_A_Backoff_Start] -> Logical6/1
  Ctrl/3(Num Slots Load) -> Num Slots/1, Gateway Out3/1, Logical3/1
  Logical3/1 -> Num Slots/4
  Logical2/1 -> Num Slots/3
  Logical1/1 -> Logical3/2
  [Slot_Done] -> Logical1/1
  Inverter/1 -> Register/1, Logical1/4
  Gateway Out/1 -> Backoff/1  "BO Start"
  Gateway Out1/1 -> Backoff/2  "BO Done"
  Gateway Out2/1 -> Backoff/3  "Idle for DIFS"
  Gateway Out3/1 -> Backoff/4  "BO Counter Load"
  Gateway Out4/1 -> Backoff/5  "BO Counter"
  Ctrl/1(BO Done) -> Backoff Done/1, Gateway Out1/1
  Register/1 -> Register1/1
  Register1/1 -> dbg_Backoff_A_active/1
  [GLOBAL_RESET] -> Logical2/1
  [reg_Force_Reset_A_Backoff] -> Logical2/2
  [Status_Tx_C_Pending] -> Inverter1/1
  Inverter1/1 -> Logical1/2
  [reg_Pause_A_Backoff] -> Inverter2/1
  Inverter2/1 -> Logical1/3

== system wlan_mac_hw/Tx Control A/Capture MAC-PHY Params ==
  Capt : Inport
  Register{1..3,6..10} (8 alike) : xbsIndex_r4/Register  init=0  rst=off  en=on  dbl_ovrd=off  block_type=register
  tag scope: Tx_A_Num_BO_Slots=global, Tx_A_Param_TxAntMask=global, Tx_A_Param_TxGain_A=global, Tx_A_Param_TxGain_B=global, Tx_A_Param_TxGain_C=global, Tx_A_Param_TxGain_D=global, Tx_A_Param_Tx_PHY_Mode=global, Tx_A_PktBuf=global
  wires:
  Register10/1 -> [Tx_A_Param_TxGain_D]
  Register9/1 -> [Tx_A_Param_TxGain_C]
  Register8/1 -> [Tx_A_Param_TxGain_B]
  [reg_Tx_A_Param_TxGain_RFD] -> Register10/1
  [reg_Tx_A_Param_TxGain_RFC] -> Register9/1
  [reg_Tx_A_Param_TxGain_RFB] -> Register8/1
  Register7/1 -> [Tx_A_Param_TxAntMask]
  [reg_Tx_A_Param_TxAntMask] -> Register7/1
  Register6/1 -> [Tx_A_Param_TxGain_A]
  [reg_Tx_A_Param_TxGain_RFA] -> Register6/1
  Register2/1 -> [Tx_A_PktBuf]
  [reg_Tx_A_Param_PktBuf] -> Register2/1
  Register3/1 -> [Tx_A_Num_BO_Slots]
  [reg_Tx_A_Param_BO_Slots] -> Register3/1
  Capt/1 -> Register2/2, Register3/2, Register6/2, Register8/2, Register9/2, Register10/2, Register7/2, Register1/2
  Register1/1 -> [Tx_A_Param_Tx_PHY_Mode]
  [reg_Tx_A_Param_PHY_Mode] -> Register1/1

== system wlan_mac_hw/Tx Control A/Posedge1 ==
  note: Rising Edge Detection
  D : Inport
  Delay : xbsIndex_r4/Delay  rst=off  infoeditControl=Selection of Reset will increase slice count due to use of real FFs and instead of SRLs  en=off  latency=1  dbl_ovrd=off  reg_retiming=off  block_type=delay
      settings: infoedit=Hardware notes: A delay line is a chain, each link of which is an SRL16 followed by a flip-flop. If register retiming is enabled, the delay line is a chain of flip-flops.  xl_area=[1 1 0 0 0 0 0]  block_version=VER_STRING_GOES_HERE
  Inverter : xbsIndex_r4/Inverter  en=off  latency=0  dbl_ovrd=off  block_type=inv
      settings: xl_area=[0 0 0 0 0 0 0]  block_version=VER_STRING_GOES_HERE
  Logical1 : xbsIndex_r4/Logical  logical_function=AND  inputs=2  en=off  latency=0  precision=Full  arith_type=Unsigned  n_bits=8  bin_pt=2  align_bp=on  dbl_ovrd=off  block_type=logical
      settings: xl_area=[1 0 0 1 0 0 0]  block_version=VER_STRING_GOES_HERE
  Q : Outport
  wires:
  Delay/1 -> Inverter/1
  Inverter/1 -> Logical1/1
  Logical1/1 -> Q/1
  D/1 -> Delay/1, Logical1/2

== system wlan_mac_hw/Tx Control A/Posedge2 ==
  note: Rising Edge Detection
  D : Inport
  Delay : xbsIndex_r4/Delay  rst=off  infoeditControl=Selection of Reset will increase slice count due to use of real FFs and instead of SRLs  en=off  latency=1  dbl_ovrd=off  reg_retiming=off  block_type=delay
      settings: infoedit=Hardware notes: A delay line is a chain, each link of which is an SRL16 followed by a flip-flop. If register retiming is enabled, the delay line is a chain of flip-flops.  xl_area=[1 1 0 0 0 0 0]  block_version=VER_STRING_GOES_HERE
  Inverter : xbsIndex_r4/Inverter  en=off  latency=0  dbl_ovrd=off  block_type=inv
      settings: xl_area=[0 0 0 0 0 0 0]  block_version=VER_STRING_GOES_HERE
  Logical1 : xbsIndex_r4/Logical  logical_function=AND  inputs=2  en=off  latency=0  precision=Full  arith_type=Unsigned  n_bits=8  bin_pt=2  align_bp=on  dbl_ovrd=off  block_type=logical
      settings: xl_area=[1 0 0 1 0 0 0]  block_version=VER_STRING_GOES_HERE
  Q : Outport
  wires:
  D/1 -> Logical1/2, Delay/1
  Logical1/1 -> Q/1
  Inverter/1 -> Logical1/1
  Delay/1 -> Inverter/1

== system wlan_mac_hw/Tx Control A/S-R Latch1 ==
  S : Inport
  R : Inport  Port=2
  Constant1 : xbsIndex_r4/Constant  const=1  gui_display_data_type=Boolean  arith_type=Boolean  n_bits=1  bin_pt=0  preci_type=Single  exp_width=8  frac_width=24  explicit_period=off  period=1  equ=P=C  opselect=C  inp2=PCIN>>17  opr=+  inp1=P  carry=CIN  dbl_ovrd=off  block_type=constant
      settings: block_version=VER_STRING_GOES_HERE
  Register2 : xbsIndex_r4/Register  init=0  rst=on  en=on  dbl_ovrd=off  block_type=register
      settings: xl_area=[1 1 0 0 0 0 0]  block_version=VER_STRING_GOES_HERE
  Q : Outport
  wires:
  S/1 -> Register2/3
  Register2/1 -> Q/1
  R/1 -> Register2/2
  Constant1/1 -> Register2/1

== system wlan_mac_hw/Tx Control A/S-R Latch2 ==
  S : Inport
  R : Inport  Port=2
  Constant1 : xbsIndex_r4/Constant  const=1  gui_display_data_type=Boolean  arith_type=Boolean  n_bits=1  bin_pt=0  preci_type=Single  exp_width=8  frac_width=24  explicit_period=off  period=1  equ=P=C  opselect=C  inp2=PCIN>>17  opr=+  inp1=P  carry=CIN  dbl_ovrd=off  block_type=constant
      settings: block_version=VER_STRING_GOES_HERE
  Register2 : xbsIndex_r4/Register  init=0  rst=on  en=on  dbl_ovrd=off  block_type=register
      settings: xl_area=[1 1 0 0 0 0 0]  block_version=VER_STRING_GOES_HERE
  Q : Outport
  wires:
  Constant1/1 -> Register2/1
  R/1 -> Register2/2
  Register2/1 -> Q/1
  S/1 -> Register2/3

== system wlan_mac_hw/Tx Control A/S-R Latch3 ==
  S : Inport
  R : Inport  Port=2
  Constant1 : xbsIndex_r4/Constant  const=1  gui_display_data_type=Boolean  arith_type=Boolean  n_bits=1  bin_pt=0  preci_type=Single  exp_width=8  frac_width=24  explicit_period=off  period=1  equ=P=C  opselect=C  inp2=PCIN>>17  opr=+  inp1=P  carry=CIN  dbl_ovrd=off  block_type=constant
      settings: block_version=VER_STRING_GOES_HERE
  Register2 : xbsIndex_r4/Register  init=0  rst=on  en=on  dbl_ovrd=off  block_type=register
      settings: xl_area=[1 1 0 0 0 0 0]  block_version=VER_STRING_GOES_HERE
  Q : Outport
  wires:
  Constant1/1 -> Register2/1
  R/1 -> Register2/2
  Register2/1 -> Q/1
  S/1 -> Register2/3

== system wlan_mac_hw/Tx Control B/Capture MAC-PHY Params ==
  Capt : Inport
  Register{1..2,6..10} (7 alike) : xbsIndex_r4/Register  init=0  rst=off  en=on  dbl_ovrd=off  block_type=register
  tag scope: Tx_B_Param_TxAntMask=global, Tx_B_Param_TxGain_A=global, Tx_B_Param_TxGain_B=global, Tx_B_Param_TxGain_C=global, Tx_B_Param_TxGain_D=global, Tx_B_Param_Tx_PHY_Mode=global, Tx_B_PktBuf=global
  wires:
  Register10/1 -> [Tx_B_Param_TxGain_D]
  Register9/1 -> [Tx_B_Param_TxGain_C]
  Register8/1 -> [Tx_B_Param_TxGain_B]
  [reg_Tx_B_Param_TxGain_RFD] -> Register10/1
  [reg_Tx_B_Param_TxGain_RFC] -> Register9/1
  [reg_Tx_B_Param_TxGain_RFB] -> Register8/1
  Register7/1 -> [Tx_B_Param_TxAntMask]
  [reg_Tx_B_Param_TxAntMask] -> Register7/1
  Register6/1 -> [Tx_B_Param_TxGain_A]
  [reg_Tx_B_Param_TxGain_RFA] -> Register6/1
  Register2/1 -> [Tx_B_PktBuf]
  [reg_Tx_B_Param_PktBuf] -> Register2/1
  Capt/1 -> Register2/2, Register6/2, Register8/2, Register9/2, Register10/2, Register7/2, Register1/2
  Register1/1 -> [Tx_B_Param_Tx_PHY_Mode]
  [reg_Tx_B_Param_PHY_Mode] -> Register1/1

== system wlan_mac_hw/Tx Control B/Posedge1 ==
  note: Rising Edge Detection
  D : Inport
  Delay : xbsIndex_r4/Delay  rst=off  infoeditControl=Selection of Reset will increase slice count due to use of real FFs and instead of SRLs  en=off  latency=1  dbl_ovrd=off  reg_retiming=off  block_type=delay
      settings: infoedit=Hardware notes: A delay line is a chain, each link of which is an SRL16 followed by a flip-flop. If register retiming is enabled, the delay line is a chain of flip-flops.  xl_area=[1 1 0 0 0 0 0]  block_version=VER_STRING_GOES_HERE
  Inverter : xbsIndex_r4/Inverter  en=off  latency=0  dbl_ovrd=off  block_type=inv
      settings: xl_area=[0 0 0 0 0 0 0]  block_version=VER_STRING_GOES_HERE
  Logical1 : xbsIndex_r4/Logical  logical_function=AND  inputs=2  en=off  latency=0  precision=Full  arith_type=Unsigned  n_bits=8  bin_pt=2  align_bp=on  dbl_ovrd=off  block_type=logical
      settings: xl_area=[1 0 0 1 0 0 0]  block_version=VER_STRING_GOES_HERE
  Q : Outport
  wires:
  D/1 -> Logical1/2, Delay/1
  Logical1/1 -> Q/1
  Inverter/1 -> Logical1/1
  Delay/1 -> Inverter/1

== system wlan_mac_hw/Tx Control B/Posedge2 ==
  note: Rising Edge Detection
  D : Inport
  Delay : xbsIndex_r4/Delay  rst=off  infoeditControl=Selection of Reset will increase slice count due to use of real FFs and instead of SRLs  en=off  latency=1  dbl_ovrd=off  reg_retiming=off  block_type=delay
      settings: infoedit=Hardware notes: A delay line is a chain, each link of which is an SRL16 followed by a flip-flop. If register retiming is enabled, the delay line is a chain of flip-flops.  xl_area=[1 1 0 0 0 0 0]  block_version=VER_STRING_GOES_HERE
  Inverter : xbsIndex_r4/Inverter  en=off  latency=0  dbl_ovrd=off  block_type=inv
      settings: xl_area=[0 0 0 0 0 0 0]  block_version=VER_STRING_GOES_HERE
  Logical1 : xbsIndex_r4/Logical  logical_function=AND  inputs=2  en=off  latency=0  precision=Full  arith_type=Unsigned  n_bits=8  bin_pt=2  align_bp=on  dbl_ovrd=off  block_type=logical
      settings: xl_area=[1 0 0 1 0 0 0]  block_version=VER_STRING_GOES_HERE
  Q : Outport
  wires:
  Delay/1 -> Inverter/1
  Inverter/1 -> Logical1/1
  Logical1/1 -> Q/1
  D/1 -> Delay/1, Logical1/2

== system wlan_mac_hw/Tx Control B/S-R Latch1 ==
  S : Inport
  R : Inport  Port=2
  Constant1 : xbsIndex_r4/Constant  const=1  gui_display_data_type=Boolean  arith_type=Boolean  n_bits=1  bin_pt=0  preci_type=Single  exp_width=8  frac_width=24  explicit_period=off  period=1  equ=P=C  opselect=C  inp2=PCIN>>17  opr=+  inp1=P  carry=CIN  dbl_ovrd=off  block_type=constant
      settings: block_version=VER_STRING_GOES_HERE
  Register2 : xbsIndex_r4/Register  init=0  rst=on  en=on  dbl_ovrd=off  block_type=register
      settings: xl_area=[1 1 0 0 0 0 0]  block_version=VER_STRING_GOES_HERE
  Q : Outport
  wires:
  Constant1/1 -> Register2/1
  R/1 -> Register2/2
  Register2/1 -> Q/1
  S/1 -> Register2/3

== system wlan_mac_hw/Tx Control B/S-R Latch2 ==
  S : Inport
  R : Inport  Port=2
  Constant1 : xbsIndex_r4/Constant  const=1  gui_display_data_type=Boolean  arith_type=Boolean  n_bits=1  bin_pt=0  preci_type=Single  exp_width=8  frac_width=24  explicit_period=off  period=1  equ=P=C  opselect=C  inp2=PCIN>>17  opr=+  inp1=P  carry=CIN  dbl_ovrd=off  block_type=constant
      settings: block_version=VER_STRING_GOES_HERE
  Register2 : xbsIndex_r4/Register  init=0  rst=on  en=on  dbl_ovrd=off  block_type=register
      settings: xl_area=[1 1 0 0 0 0 0]  block_version=VER_STRING_GOES_HERE
  Q : Outport
  wires:
  S/1 -> Register2/3
  Register2/1 -> Q/1
  R/1 -> Register2/2
  Constant1/1 -> Register2/1

== system wlan_mac_hw/Tx Control C/C Backoff ==
  note: Sanity Checks:
      | Assuming IDLE_FOR_DIFS asserts and stays high.
      |
      | If NUM_BO_SLOTS = 0, core should transmit when BACKOFF_START asserts with no extra waiting
      |
      | If NUM_BO_SLOTS = 1, core should transmit exactly 1 slot time after BACKOFF_START asserts
  note: Software-initiated backoff gets priority
      | But any "start backoff" is ignored if a
      | previous backoff is still active.
  Reset : Inport
  Backoff : Scope  NumInputPorts=5
      settings: YMin=-1~0.95~0.95~-5~-5  YMax=1~1.05~1.05~5~5
  Constant : xbsIndex_r4/Constant  const=0  gui_display_data_type=Fixed-point  arith_type=Unsigned  n_bits=1  bin_pt=0  preci_type=Single  exp_width=8  frac_width=24  explicit_period=off  period=1  equ=P=C  opselect=C  inp2=PCIN>>17  opr=+  inp1=P  carry=CIN  dbl_ovrd=off  block_type=constant
  Convert : xbsIndex_r4/Convert  gui_display_data_type=Fixed-point  arith_type=Unsigned  n_bits=NB_CNTR_NUM_SLOTS  bin_pt=0  float_type=Single  exp_bits=8  fraction_bits=24  quantization=Truncate  overflow=Wrap  en=off  latency=0  dbl_ovrd=off  pipeline=off  block_type=convert
  Ctrl : Subsystem
  Gateway Out{,1..4} (5 alike) : xbsIndex_r4/Gateway Out  inherit_from_input=off  hdl_port=off  timing_constraint=None  locs_specified=off  LOCs={}  UseAsDAC=off  DACChannel='1'  block_type=gatewayout
  Inverter : xbsIndex_r4/Inverter  en=off  latency=0  dbl_ovrd=off  block_type=inv
      settings: xl_area=[0 0 0 0 0 0 0]  block_version=VER_STRING_GOES_HERE
  Logical1 : xbsIndex_r4/Logical  logical_function=AND  inputs=2  en=off  latency=0  precision=Full  arith_type=Unsigned  n_bits=16  bin_pt=0  align_bp=on  dbl_ovrd=off  block_type=logical
  Logical2 : xbsIndex_r4/Logical  logical_function=OR  inputs=2  en=off  latency=0  precision=Full  arith_type=Unsigned  n_bits=16  bin_pt=0  align_bp=on  dbl_ovrd=off  block_type=logical
  Logical3 : xbsIndex_r4/Logical  logical_function=OR  inputs=2  en=off  latency=0  precision=Full  arith_type=Unsigned  n_bits=16  bin_pt=0  align_bp=on  dbl_ovrd=off  block_type=logical
  Num Slots : xbsIndex_r4/Counter  cnt_type=Free Running  cnt_to=0  operation=Down  start_count=0  cnt_by_val=1  arith_type=Unsigned  n_bits=NB_CNTR_NUM_SLOTS  bin_pt=0  load_pin=on  rst=on  en=on  explicit_period=off  period=1  dbl_ovrd=off  use_behavioral_HDL=off  implementation=Fabric  block_type=counter
  Register : xbsIndex_r4/Register  init=0  rst=off  en=off  dbl_ovrd=off  block_type=register
  Register1 : xbsIndex_r4/Register  init=0  rst=off  en=off  dbl_ovrd=off  block_type=register
  Register2 : xbsIndex_r4/Register  init=0  rst=off  en=on  dbl_ovrd=off  block_type=register
      settings: xl_area=[1 1 0 0 0 0 0]  block_version=VER_STRING_GOES_HERE
  Relational1 : xbsIndex_r4/Relational  mode=a=b  en=off  latency=0  dbl_ovrd=off  block_type=relational
  dbg_Backoff_C_active : xbsIndex_r4/Gateway Out  inherit_from_input=off  hdl_port=on  timing_constraint=None  locs_specified=off  LOCs={}  UseAsDAC=off  DACChannel='1'  block_type=gatewayout
  Backoff Done : Outport
  tag scope: Status_Current_C_Backoff_Count=global
  wires:
  Convert/1 -> Num Slots/2
  [IDLE_FOR_TXDIFS] -> Ctrl/4(Idle for DIFS), Gateway Out2/1
  Constant/1 -> Relational1/2
  Relational1/1 -> Inverter/1, Ctrl/1(BO Zero)
  Num Slots/1 -> Relational1/1, [Status_Current_C_Backoff_Count], Gateway Out4/1
  [Tx_C_Num_BO_Slots] -> Register2/1, Ctrl/3(Num Slots)
  Register2/1 -> Convert/1
  [Tx_C_Backoff_Start] -> Register2/2, Gateway Out/1, Ctrl/2(BO Start)
  Ctrl/3(Num Slots Load) -> Num Slots/1, Gateway Out3/1, Logical3/1
  Logical3/1 -> Num Slots/4
  Logical2/1 -> Num Slots/3
  Logical1/1 -> Logical3/2
  [Slot_Done] -> Logical1/1
  Inverter/1 -> Logical1/2, Register/1
  Gateway Out/1 -> Backoff/1  "BO Start"
  Gateway Out1/1 -> Backoff/2  "BO Done"
  Gateway Out2/1 -> Backoff/3  "Idle for DIFS"
  Gateway Out3/1 -> Backoff/4  "BO Counter Load"
  Gateway Out4/1 -> Backoff/5  "BO Counter"
  Ctrl/1(BO Done) -> Backoff Done/1, Gateway Out1/1
  Register/1 -> Register1/1
  Register1/1 -> dbg_Backoff_C_active/1
  Reset/1 -> Logical2/1
  [reg_Force_Reset_C_Backoff] -> Logical2/2
